simulink model "actuators_basicIO_2024a"  (R2024a)
settings: Solver=ode2  StartTime=0.0  StopTime=inf  FixedStep=1/500  RelTol=1e-3  EnableMultiTasking=on
undefined symbols (not defined in the file): HIL
libraries: quarc_library x85, simulink x4
settings Model: ExtModeTrigDuration=10000  Creator=Lorena Gonzalez  LastModifiedBy=Lorena Gonzalez
settings SolverCC: AlgebraicLoopSolver=TrustRegion  PositivePriorityOrder=on
settings DataIOCC: ReturnWorkspaceOutputs=off
settings DebuggingCC: UnconnectedInputMsg=warning  UnconnectedOutputMsg=warning  UnconnectedLineMsg=warning  ArithmeticOperatorsInVariantConditions=warning
settings ModelReferenceCC: EnableRefExpFcnMdlSchedulingChecks=on
settings SFSimCC: SimUseLocalCustomCode=off  CustomCodeUndefinedFunction=UseInterfaceOnly
settings RTWCC: Description=QUARC Win64 Target Using Toolchain  SystemTargetFile=quarc_win64.tlc  TemplateMakefile=quarc_default_tmf  RTWUseLocalCustomCode=off  Toolchain=QUARC win64 | nmake (64-bit Windows)  BuildConfiguration=Faster Runs  GPUComputeCapability=3.5
settings CodeAppCC: StateflowObjectComments=on
settings STFCustomTargetCC: ConcurrentExecutionCompliant=on  SystemTargetFile=quarc_win64.tlc
settings GRTTargetCC: ParMdlRefBuildCompliant=off  CompOptLevelCompliant=off  CombineOutputUpdateFcns=off  MatFileLogging=off  CPPClassGenCompliant=off  GRTInterface=on  ExtMode=on  ExtModeMexFile=quarc_comm
settings ConfigComp: CovMetricSettings=dswe

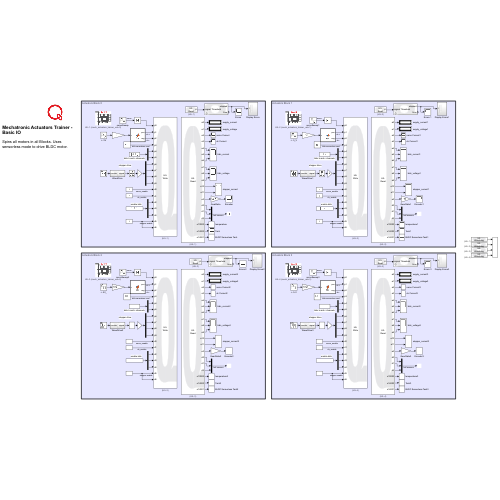
[thumbnail: Simulink's stored preview of the top-level diagram]
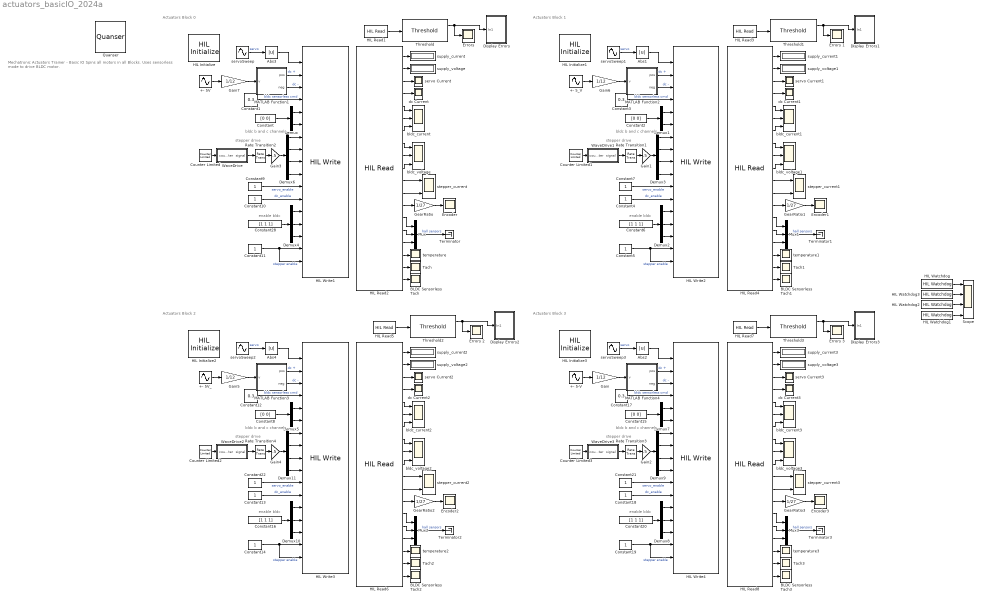
== system actuators_basicIO_2024a ==
  note: bldc b and c channels
  note: enable bldc
  note: Actuators Block 3
  note: Mechatronic Actuators Trainer - Basic IO
      |
      | Spins all motors in all Blocks. Uses sensorless mode to drive BLDC motor.
  note: bldc b and c channels
  note: stepper drive
  note: Actuators Block 0
  note: stepper drive
  note: Actuators Block 1
  note: enable bldc
  note: bldc b and c channels
  note: Actuators Block 2
  note: enable bldc
  note: stepper drive
  note: bldc b and c channels
  note: stepper drive
  note: enable bldc
  +- 5-V : Sin  Amplitude=5  Frequency=.75  SampleTime=0
  +- 5V : Sin  Amplitude=5  Frequency=.75  SampleTime=0
  +- 5V_ : Sin  Amplitude=5  Frequency=.75  SampleTime=0
  +- 5_V : Sin  Amplitude=5  Frequency=.75  SampleTime=0
  Abs{1..4} (4 alike) : Abs  SaturateOnIntegerOverflow=off
  BLDC Sensorless Tach{,1..3} (4 alike) : Scope
  Constant{,2,8,15} (4 alike) : Constant  Value=[0 0]
  Constant{1,3,12,17} (4 alike) : Constant  Value=0.3
  Constant{4..5,7,9..11,13..14,18..19,21..22} (12 alike) : Constant
  Constant{6,16,20,28} (4 alike) : Constant  Value=[1 1 1]
  Counter Limited{,1..3} (4 alike) : simulink/Sources/Counter Limited  uplimit=3  tsamp=1/100
  Demux{,1,5,7} (4 alike) : Demux  Outputs=2
  Demux{2,4,8,10} (4 alike) : Demux  Outputs=3
  Demux{3,6,9,11} (4 alike) : Demux
  Display Errors : Subsystem
  Display Errors1 : Subsystem
  Display Errors2 : Subsystem
  Display Errors3 : Subsystem
  Encoder{,1..3} (4 alike) : Scope
  Errors {,1..3} (4 alike) : Scope
  Gain{,5..7} (4 alike) : Gain  Gain=1/12
  Gain{1..4} (4 alike) : Gain  Gain=.5
  GearRatio{,1..3} (4 alike) : Gain  Gain=1/27
  HIL Initialize : quarc_library/Data Acquisition/Generic/Configuration/HIL Initialize  object_name=HIL-1  board_type=mech_actuators_trainer_usb  board_number=0  board_options=supply_voltage_low_limit=10.0;supply_voltage_high_limit=16.0;supply_current_high_limit=8.0;dc_motor_current_high_limit=1.1;servo_motor_current_high_limit=1.3;bldc_motor_current_high_limit=2.0;stepper_motor_current_high_limit=1.7;servo_pwm_range=0;enc_dir=0;bldc_motor_mode=1;bldc_start_tc=0.03;bldc_start_target=1200  exclusive=off  active=on  hardware_clocks=[0]  clock_modes=[]  initial_clock_frequencies=[]  set_clock_params_at_start=off  set_clock_params_at_switch_in=off  set_clock_frequencies_at_start=off  set_clock_frequencies_at_switch_in=off  analog_input_channels=[0:11]  analog_input_configurations=[]  analog_input_maximums=3  analog_input_minimums=-3  set_analog_input_params_at_start=off  set_analog_input_params_at_switch_in=off  analog_output_channels=[]  analog_output_maximums=[]  analog_output_minimums=[]  initial_analog_outputs=[]  final_analog_outputs=[]  watchdog_analog_outputs=[]  set_analog_output_params_at_start=off  set_analog_output_params_at_switch_in=off  set_analog_outputs_at_start=off  set_analog_outputs_at_switch_in=off  set_analog_outputs_at_terminate=off  set_analog_outputs_at_switch_out=off  set_analog_outputs_on_watchdog=off  digital_input_channels=[0:17]  digital_output_channels=[0:6]  digital_output_configuration=[]  initial_digital_outputs=[1]  final_digital_outputs=[0]  watchdog_digital_outputs=[0]  set_digital_output_params_at_start=off  set_digital_output_params_at_switch_in=off  set_digital_outputs_at_start=on  set_digital_outputs_at_switch_in=off  set_digital_outputs_at_terminate=on  set_digital_outputs_at_switch_out=off  set_digital_outputs_on_watchdog=on  encoder_channels=[0]  quadrature=[4]  encoder_filter_frequency=[]  initial_encoder_counts=[0]  set_encoder_params_at_start=on  set_encoder_params_at_switch_in=off  set_encoder_counts_at_start=on  set_encoder_counts_at_switch_in=off  pwm_channels=[0:9]  pwm_modes=[0]  pwm_frequency=23195  pwm_configuration=[1]  pwm_alignment=[0]  pwm_polarity=[1]  pwm_leading_deadband=[0]  pwm_trailing_deadband=[0]  initial_pwm_outputs=[0]  final_pwm_outputs=[0]  watchdog_pwm_outputs=[0]  set_pwm_params_at_start=off  set_pwm_params_at_switch_in=off  set_pwm_outputs_at_start=on  set_pwm_outputs_at_switch_in=off  set_pwm_outputs_at_terminate=on  set_pwm_outputs_at_switch_out=off  set_pwm_outputs_on_watchdog=on  other_output_channels=[]  initial_other_outputs=[]  final_other_outputs=[]  watchdog_other_outputs=[]  set_other_outputs_at_start=off  set_other_outputs_at_switch_in=off  set_other_outputs_at_terminate=off  set_other_outputs_at_switch_out=off  set_other_outputs_on_watchdog=off
  HIL Initialize1 : quarc_library/Data Acquisition/Generic/Configuration/HIL Initialize  object_name=HIL-2  board_type=mech_actuators_trainer_usb  board_number=1  board_options=supply_voltage_low_limit=10.0;supply_voltage_high_limit=16.0;supply_current_high_limit=8.0;dc_motor_current_high_limit=1.1;servo_motor_current_high_limit=1.3;bldc_motor_current_high_limit=2.0;stepper_motor_current_high_limit=1.7;servo_pwm_range=0;enc_dir=0;bldc_motor_mode=1;bldc_start_tc=0.03;bldc_start_target=1200  exclusive=off  active=on  hardware_clocks=[0]  clock_modes=[]  initial_clock_frequencies=[]  set_clock_params_at_start=off  set_clock_params_at_switch_in=off  set_clock_frequencies_at_start=off  set_clock_frequencies_at_switch_in=off  analog_input_channels=[0:11]  analog_input_configurations=[]  analog_input_maximums=3  analog_input_minimums=-3  set_analog_input_params_at_start=off  set_analog_input_params_at_switch_in=off  analog_output_channels=[]  analog_output_maximums=[]  analog_output_minimums=[]  initial_analog_outputs=[]  final_analog_outputs=[]  watchdog_analog_outputs=[]  set_analog_output_params_at_start=off  set_analog_output_params_at_switch_in=off  set_analog_outputs_at_start=off  set_analog_outputs_at_switch_in=off  set_analog_outputs_at_terminate=off  set_analog_outputs_at_switch_out=off  set_analog_outputs_on_watchdog=off  digital_input_channels=[0:17]  digital_output_channels=[0:6]  digital_output_configuration=[]  initial_digital_outputs=[1]  final_digital_outputs=[0]  watchdog_digital_outputs=[0]  set_digital_output_params_at_start=off  set_digital_output_params_at_switch_in=off  set_digital_outputs_at_start=on  set_digital_outputs_at_switch_in=off  set_digital_outputs_at_terminate=on  set_digital_outputs_at_switch_out=off  set_digital_outputs_on_watchdog=on  encoder_channels=[0]  quadrature=[4]  encoder_filter_frequency=[]  initial_encoder_counts=[0]  set_encoder_params_at_start=on  set_encoder_params_at_switch_in=off  set_encoder_counts_at_start=on  set_encoder_counts_at_switch_in=off  pwm_channels=[0:9]  pwm_modes=[0]  pwm_frequency=23195  pwm_configuration=[1]  pwm_alignment=[0]  pwm_polarity=[1]  pwm_leading_deadband=[0]  pwm_trailing_deadband=[0]  initial_pwm_outputs=[0]  final_pwm_outputs=[0]  watchdog_pwm_outputs=[0]  set_pwm_params_at_start=off  set_pwm_params_at_switch_in=off  set_pwm_outputs_at_start=on  set_pwm_outputs_at_switch_in=off  set_pwm_outputs_at_terminate=on  set_pwm_outputs_at_switch_out=off  set_pwm_outputs_on_watchdog=on  other_output_channels=[]  initial_other_outputs=[]  final_other_outputs=[]  watchdog_other_outputs=[]  set_other_outputs_at_start=off  set_other_outputs_at_switch_in=off  set_other_outputs_at_terminate=off  set_other_outputs_at_switch_out=off  set_other_outputs_on_watchdog=off
  HIL Initialize2 : quarc_library/Data Acquisition/Generic/Configuration/HIL Initialize  object_name=HIL-3  board_type=mech_actuators_trainer_usb  board_number=2  board_options=supply_voltage_low_limit=10.0;supply_voltage_high_limit=16.0;supply_current_high_limit=8.0;dc_motor_current_high_limit=1.1;servo_motor_current_high_limit=1.3;bldc_motor_current_high_limit=2.0;stepper_motor_current_high_limit=1.7;servo_pwm_range=0;enc_dir=0;bldc_motor_mode=1;bldc_start_tc=0.03;bldc_start_target=1200  exclusive=off  active=on  hardware_clocks=[0]  clock_modes=[]  initial_clock_frequencies=[]  set_clock_params_at_start=off  set_clock_params_at_switch_in=off  set_clock_frequencies_at_start=off  set_clock_frequencies_at_switch_in=off  analog_input_channels=[0:11]  analog_input_configurations=[]  analog_input_maximums=3  analog_input_minimums=-3  set_analog_input_params_at_start=off  set_analog_input_params_at_switch_in=off  analog_output_channels=[]  analog_output_maximums=[]  analog_output_minimums=[]  initial_analog_outputs=[]  final_analog_outputs=[]  watchdog_analog_outputs=[]  set_analog_output_params_at_start=off  set_analog_output_params_at_switch_in=off  set_analog_outputs_at_start=off  set_analog_outputs_at_switch_in=off  set_analog_outputs_at_terminate=off  set_analog_outputs_at_switch_out=off  set_analog_outputs_on_watchdog=off  digital_input_channels=[0:17]  digital_output_channels=[0:6]  digital_output_configuration=[]  initial_digital_outputs=[1]  final_digital_outputs=[0]  watchdog_digital_outputs=[0]  set_digital_output_params_at_start=off  set_digital_output_params_at_switch_in=off  set_digital_outputs_at_start=on  set_digital_outputs_at_switch_in=off  set_digital_outputs_at_terminate=on  set_digital_outputs_at_switch_out=off  set_digital_outputs_on_watchdog=on  encoder_channels=[0]  quadrature=[4]  encoder_filter_frequency=[]  initial_encoder_counts=[0]  set_encoder_params_at_start=on  set_encoder_params_at_switch_in=off  set_encoder_counts_at_start=on  set_encoder_counts_at_switch_in=off  pwm_channels=[0:9]  pwm_modes=[0]  pwm_frequency=23195  pwm_configuration=[1]  pwm_alignment=[0]  pwm_polarity=[1]  pwm_leading_deadband=[0]  pwm_trailing_deadband=[0]  initial_pwm_outputs=[0]  final_pwm_outputs=[0]  watchdog_pwm_outputs=[0]  set_pwm_params_at_start=off  set_pwm_params_at_switch_in=off  set_pwm_outputs_at_start=on  set_pwm_outputs_at_switch_in=off  set_pwm_outputs_at_terminate=on  set_pwm_outputs_at_switch_out=off  set_pwm_outputs_on_watchdog=on  other_output_channels=[]  initial_other_outputs=[]  final_other_outputs=[]  watchdog_other_outputs=[]  set_other_outputs_at_start=off  set_other_outputs_at_switch_in=off  set_other_outputs_at_terminate=off  set_other_outputs_at_switch_out=off  set_other_outputs_on_watchdog=off
  HIL Initialize3 : quarc_library/Data Acquisition/Generic/Configuration/HIL Initialize  object_name=HIL-4  board_type=mech_actuators_trainer_usb  board_number=3  board_options=supply_voltage_low_limit=10.0;supply_voltage_high_limit=16.0;supply_current_high_limit=8.0;dc_motor_current_high_limit=1.1;servo_motor_current_high_limit=1.3;bldc_motor_current_high_limit=2.0;stepper_motor_current_high_limit=1.7;servo_pwm_range=0;enc_dir=0;bldc_motor_mode=1;bldc_start_tc=0.03;bldc_start_target=1200  exclusive=off  active=on  hardware_clocks=[0]  clock_modes=[]  initial_clock_frequencies=[]  set_clock_params_at_start=off  set_clock_params_at_switch_in=off  set_clock_frequencies_at_start=off  set_clock_frequencies_at_switch_in=off  analog_input_channels=[0:11]  analog_input_configurations=[]  analog_input_maximums=3  analog_input_minimums=-3  set_analog_input_params_at_start=off  set_analog_input_params_at_switch_in=off  analog_output_channels=[]  analog_output_maximums=[]  analog_output_minimums=[]  initial_analog_outputs=[]  final_analog_outputs=[]  watchdog_analog_outputs=[]  set_analog_output_params_at_start=off  set_analog_output_params_at_switch_in=off  set_analog_outputs_at_start=off  set_analog_outputs_at_switch_in=off  set_analog_outputs_at_terminate=off  set_analog_outputs_at_switch_out=off  set_analog_outputs_on_watchdog=off  digital_input_channels=[0:17]  digital_output_channels=[0:6]  digital_output_configuration=[]  initial_digital_outputs=[1]  final_digital_outputs=[0]  watchdog_digital_outputs=[0]  set_digital_output_params_at_start=off  set_digital_output_params_at_switch_in=off  set_digital_outputs_at_start=on  set_digital_outputs_at_switch_in=off  set_digital_outputs_at_terminate=on  set_digital_outputs_at_switch_out=off  set_digital_outputs_on_watchdog=on  encoder_channels=[0]  quadrature=[4]  encoder_filter_frequency=[]  initial_encoder_counts=[0]  set_encoder_params_at_start=on  set_encoder_params_at_switch_in=off  set_encoder_counts_at_start=on  set_encoder_counts_at_switch_in=off  pwm_channels=[0:9]  pwm_modes=[0]  pwm_frequency=23195  pwm_configuration=[1]  pwm_alignment=[0]  pwm_polarity=[1]  pwm_leading_deadband=[0]  pwm_trailing_deadband=[0]  initial_pwm_outputs=[0]  final_pwm_outputs=[0]  watchdog_pwm_outputs=[0]  set_pwm_params_at_start=off  set_pwm_params_at_switch_in=off  set_pwm_outputs_at_start=on  set_pwm_outputs_at_switch_in=off  set_pwm_outputs_at_terminate=on  set_pwm_outputs_at_switch_out=off  set_pwm_outputs_on_watchdog=on  other_output_channels=[]  initial_other_outputs=[]  final_other_outputs=[]  watchdog_other_outputs=[]  set_other_outputs_at_start=off  set_other_outputs_at_switch_in=off  set_other_outputs_at_terminate=off  set_other_outputs_at_switch_out=off  set_other_outputs_on_watchdog=off
  HIL Read1 : quarc_library/Data Acquisition/Generic/Immediate I//O/HIL Read  object_name=HIL-1  analog_channels=[]  encoder_channels=[]  digital_channels=[3:17]  other_channels=[]  sample_time=qc_get_step_size  active=on  vector_output=on  data_type_mode=Inherit via back propagation  encoder_data_type=double  digital_data_type=boolean
  HIL Read2 : quarc_library/Data Acquisition/Generic/Immediate I//O/HIL Read  object_name=HIL-1  analog_channels=[0:11]  encoder_channels=[0]  digital_channels=[0:2]  other_channels=[10000 14000:14001]  sample_time=qc_get_step_size  active=on  vector_output=off  data_type_mode=Inherit via back propagation  encoder_data_type=double  digital_data_type=boolean
  HIL Read3 : quarc_library/Data Acquisition/Generic/Immediate I//O/HIL Read  object_name=HIL-2  analog_channels=[]  encoder_channels=[]  digital_channels=[3:17]  other_channels=[]  sample_time=qc_get_step_size  active=on  vector_output=on  data_type_mode=Inherit via back propagation  encoder_data_type=double  digital_data_type=boolean
  HIL Read4 : quarc_library/Data Acquisition/Generic/Immediate I//O/HIL Read  object_name=HIL-2  analog_channels=[0:11]  encoder_channels=[0]  digital_channels=[0:2]  other_channels=[10000 14000:14001]  sample_time=qc_get_step_size  active=on  vector_output=off  data_type_mode=Inherit via back propagation  encoder_data_type=double  digital_data_type=boolean
  HIL Read5 : quarc_library/Data Acquisition/Generic/Immediate I//O/HIL Read  object_name=HIL-3  analog_channels=[]  encoder_channels=[]  digital_channels=[3:17]  other_channels=[]  sample_time=qc_get_step_size  active=on  vector_output=on  data_type_mode=Inherit via back propagation  encoder_data_type=double  digital_data_type=boolean
  HIL Read6 : quarc_library/Data Acquisition/Generic/Immediate I//O/HIL Read  object_name=HIL-3  analog_channels=[0:11]  encoder_channels=[0]  digital_channels=[0:2]  other_channels=[10000 14000:14001]  sample_time=qc_get_step_size  active=on  vector_output=off  data_type_mode=Inherit via back propagation  encoder_data_type=double  digital_data_type=boolean
  HIL Read7 : quarc_library/Data Acquisition/Generic/Immediate I//O/HIL Read  object_name=HIL-4  analog_channels=[]  encoder_channels=[]  digital_channels=[3:17]  other_channels=[]  sample_time=qc_get_step_size  active=on  vector_output=on  data_type_mode=Inherit via back propagation  encoder_data_type=double  digital_data_type=boolean
  HIL Read8 : quarc_library/Data Acquisition/Generic/Immediate I//O/HIL Read  object_name=HIL-4  analog_channels=[0:11]  encoder_channels=[0]  digital_channels=[0:2]  other_channels=[10000 14000:14001]  sample_time=qc_get_step_size  active=on  vector_output=off  data_type_mode=Inherit via back propagation  encoder_data_type=double  digital_data_type=boolean
  HIL Watchdog : quarc_library/Data Acquisition/Generic/Watchdog/HIL Watchdog  object_name=HIL-1  timeout=0.1  sample_time=qc_get_step_size  active=off
      settings: AttributesFormatString=(%<object_name>)  SourceProductName=QUARC Targets
  HIL Watchdog1 : quarc_library/Data Acquisition/Generic/Watchdog/HIL Watchdog  object_name=HIL-4  timeout=0.1  sample_time=qc_get_step_size  active=off
      settings: AttributesFormatString=(%<object_name>)  SourceProductName=QUARC Targets
  HIL Watchdog2 : quarc_library/Data Acquisition/Generic/Watchdog/HIL Watchdog  object_name=HIL-3  timeout=0.1  sample_time=qc_get_step_size  active=off
      settings: AttributesFormatString=(%<object_name>)  SourceProductName=QUARC Targets
  HIL Watchdog3 : quarc_library/Data Acquisition/Generic/Watchdog/HIL Watchdog  object_name=HIL-2  timeout=0.1  sample_time=qc_get_step_size  active=off
      settings: AttributesFormatString=(%<object_name>)  SourceProductName=QUARC Targets
  HIL Write1 : quarc_library/Data Acquisition/Generic/Immediate I//O/HIL Write  object_name=HIL-1  analog_channels=[]  pwm_channels=[0:9]  digital_channels=[0:6]  other_channels=[]  sample_time=-1  active=off  vector_input=off
  HIL Write2 : quarc_library/Data Acquisition/Generic/Immediate I//O/HIL Write  object_name=HIL-2  analog_channels=[]  pwm_channels=[0:9]  digital_channels=[0:6]  other_channels=[]  sample_time=-1  active=off  vector_input=off
  HIL Write3 : quarc_library/Data Acquisition/Generic/Immediate I//O/HIL Write  object_name=HIL-3  analog_channels=[]  pwm_channels=[0:9]  digital_channels=[0:6]  other_channels=[]  sample_time=-1  active=off  vector_input=off
  HIL Write4 : quarc_library/Data Acquisition/Generic/Immediate I//O/HIL Write  object_name=HIL-4  analog_channels=[]  pwm_channels=[0:9]  digital_channels=[0:6]  other_channels=[]  sample_time=-1  active=off  vector_input=off
  MATLAB Function1 : MATLAB Function  TreatAsAtomicUnit=on
  MATLAB Function2 : MATLAB Function  TreatAsAtomicUnit=on
  MATLAB Function3 : MATLAB Function  TreatAsAtomicUnit=on
  MATLAB Function4 : MATLAB Function  TreatAsAtomicUnit=on
  Mux{,1..3} (4 alike) : Mux  Inputs=3
  Quanser : quarc_library/Logos/Quanser
  Rate Transition{1..4} (4 alike) : RateTransition
  Scope : Scope  NumInputPorts=4
  Tach{,1..3} (4 alike) : Scope
  Terminator{,1..3} (4 alike) : Terminator
  Threshold{,1..3} (4 alike) : quarc_library/Discontinuities/Threshold  operator=>  param_src=Specify via dialog  threshold=0  duration=0.02
      settings: SourceProductName=QUARC Targets
  WaveDrive : Subsystem
  WaveDrive1 : Subsystem
  WaveDrive2 : Subsystem
  WaveDrive3 : Subsystem
  bldc_current{,1..3} (4 alike) : Scope  NumInputPorts=3
  bldc_voltage{,1..3} (4 alike) : Scope  NumInputPorts=3
  dc Current{,1..3} (4 alike) : Scope
  servo Current{,1..3} (4 alike) : Scope
  servoSweep{,1..3} (4 alike) : Sin  SampleTime=0
  stepper_current{,1..3} (4 alike) : Scope  NumInputPorts=2
  supply_current{,1..3} (4 alike) : Display
  supply_voltage{,1..3} (4 alike) : Display
  temperature{,1..3} (4 alike) : Scope
  wires:
  Demux10/3 -> HIL Write3/15
  Demux11/4 -> HIL Write3/10
  HIL Read7/1 -> Threshold3/1
  HIL Read6/1 -> supply_current2/1
  HIL Read8/12 -> stepper_current3/2
  Threshold3/1 -> Display Errors3/1(In1), Errors 3/1
  HIL Read8/3 -> servo Current3/1
  HIL Read8/10 -> bldc_voltage3/3
  Rate Transition2/1 -> Gain3/1
  MATLAB Function2/2(neg) -> HIL Write2/3  "dc -"
  Gain5/1 -> MATLAB Function3/1(v)
  HIL Read8/6 -> bldc_current3/2
  HIL Read3/1 -> Threshold1/1
  HIL Read6/19 -> BLDC Sensorless Tach2/1
  HIL Read6/10 -> bldc_voltage2/3
  HIL Read5/1 -> Threshold2/1
  HIL Read4/11 -> stepper_current1/1
  Threshold1/1 -> Display Errors1/1(In1), Errors 1/1
  Threshold2/1 -> Display Errors2/1(In1), Errors 2/1
  HIL Read1/1 -> Threshold/1
  GearRatio1/1 -> Encoder1/1
  Counter Limited3/1 -> WaveDrive3/1(counter)
  Demux6/4 -> HIL Write1/10
  Constant5/1 -> HIL Write2/16, HIL Write2/17  "stepper enable"
  servoSweep2/1 -> Abs4/1  "servo"
  GearRatio3/1 -> Encoder3/1
  Constant7/1 -> HIL Write2/11  "servo_enable"
  HIL Read2/7 -> bldc_current/3
  Constant/1 -> Demux/1
  Demux9/3 -> HIL Write4/9
  Gain7/1 -> MATLAB Function1/1(v)
  Gain/1 -> MATLAB Function4/1(v)
  Demux11/2 -> HIL Write3/8
  Demux8/2 -> HIL Write4/14
  HIL Read2/11 -> stepper_current/1
  Counter Limited/1 -> WaveDrive/1(counter)
  HIL Read6/3 -> servo Current2/1
  HIL Read6/16 -> Mux2/3
  WaveDrive2/1(signal) -> Rate Transition4/1
  HIL Read8/19 -> BLDC Sensorless Tach3/1
  HIL Read8/9 -> bldc_voltage3/2
  Constant14/1 -> HIL Write3/16, HIL Write3/17  "stepper enable"
  Constant8/1 -> Demux5/1
  Demux10/2 -> HIL Write3/14
  HIL Read8/16 -> Mux3/3
  Constant13/1 -> HIL Write3/12  "dc_enable"
  HIL Read6/11 -> stepper_current2/1
  HIL Read6/12 -> stepper_current2/2
  Demux8/1 -> HIL Write4/13
  Constant10/1 -> HIL Write1/12  "dc_enable"
  HIL Read6/18 -> Tach2/1
  Constant22/1 -> HIL Write3/11  "servo_enable"
  Demux11/1 -> HIL Write3/7
  Constant15/1 -> Demux7/1
  HIL Read6/4 -> dc Current2/1
  MATLAB Function3/1(pos) -> HIL Write3/2  "dc +"
  HIL Read6/6 -> bldc_current2/2
  HIL Read4/12 -> stepper_current1/2
  Mux1/1 -> Terminator1/1  "hall sensors"
  Mux2/1 -> Terminator2/1  "hall sensors"
  HIL Read6/9 -> bldc_voltage2/2
  HIL Read6/7 -> bldc_current2/3
  HIL Read6/2 -> supply_voltage2/1
  Rate Transition4/1 -> Gain4/1
  Demux7/1 -> HIL Write4/5
  Demux8/3 -> HIL Write4/15
  Demux6/1 -> HIL Write1/7
  MATLAB Function2/1(pos) -> HIL Write2/2  "dc +"
  Gain4/1 -> Demux11/1
  Mux3/1 -> Terminator3/1  "hall sensors"
  HIL Read6/8 -> bldc_voltage2/1
  Demux9/4 -> HIL Write4/10
  MATLAB Function3/2(neg) -> HIL Write3/3  "dc -"
  Counter Limited1/1 -> WaveDrive1/1(counter)
  servoSweep1/1 -> Abs1/1  "servo"
  GearRatio2/1 -> Encoder2/1
  Counter Limited2/1 -> WaveDrive2/1(counter)
  HIL Read8/17 -> temperature3/1
  Demux/1 -> HIL Write1/5
  Gain2/1 -> Demux9/1
  servoSweep3/1 -> Abs2/1  "servo"
  HIL Read6/5 -> bldc_current2/1
  WaveDrive1/1(signal) -> Rate Transition1/1
  HIL Read4/16 -> Mux1/3
  Constant1/1 -> HIL Write1/4  "bldc sensorless cmd"
  Demux10/1 -> HIL Write3/13
  Abs4/1 -> HIL Write3/1
  HIL Read2/1 -> supply_current/1
  Constant12/1 -> HIL Write3/4  "bldc sensorless cmd"
  Constant16/1 -> Demux10/1
  Abs2/1 -> HIL Write4/1
  HIL Read6/17 -> temperature2/1
  Demux5/1 -> HIL Write3/5
  HIL Read4/8 -> bldc_voltage1/1
  Constant20/1 -> Demux8/1
  HIL Read8/13 -> GearRatio3/1
  WaveDrive3/1(signal) -> Rate Transition3/1
  HIL Read6/15 -> Mux2/2
  HIL Read4/3 -> servo Current1/1
  Rate Transition3/1 -> Gain2/1
  Demux7/2 -> HIL Write4/6
  HIL Read8/14 -> Mux3/1
  Demux9/1 -> HIL Write4/7
  Gain1/1 -> Demux3/1
  MATLAB Function4/1(pos) -> HIL Write4/2  "dc +"
  HIL Read8/7 -> bldc_current3/3
  Constant17/1 -> HIL Write4/4  "bldc sensorless cmd"
  HIL Read2/5 -> bldc_current/1
  Constant21/1 -> HIL Write4/11  "servo_enable"
  Demux9/2 -> HIL Write4/8
  HIL Read8/18 -> Tach3/1
  HIL Read8/4 -> dc Current3/1
  HIL Read8/8 -> bldc_voltage3/1
  HIL Read4/19 -> BLDC Sensorless Tach1/1
  Constant19/1 -> HIL Write4/16, HIL Write4/17  "stepper enable"
  HIL Read8/2 -> supply_voltage3/1
  HIL Read4/2 -> supply_voltage1/1
  HIL Read8/15 -> Mux3/2
  HIL Read4/18 -> Tach1/1
  HIL Read4/6 -> bldc_current1/2
  HIL Read4/14 -> Mux1/1
  Constant4/1 -> HIL Write2/12  "dc_enable"
  Demux2/1 -> HIL Write2/13
  HIL Read2/6 -> bldc_current/2
  HIL Read8/1 -> supply_current3/1
  HIL Read4/10 -> bldc_voltage1/3
  Rate Transition1/1 -> Gain1/1
  Demux1/2 -> HIL Write2/6
  HIL Read4/7 -> bldc_current1/3
  Demux2/2 -> HIL Write2/14
  HIL Read2/14 -> Mux/1
  Constant2/1 -> Demux1/1
  Demux11/3 -> HIL Write3/9
  HIL Read4/1 -> supply_current1/1
  MATLAB Function4/2(neg) -> HIL Write4/3  "dc -"
  HIL Read4/13 -> GearRatio1/1
  Gain6/1 -> MATLAB Function2/1(v)
  HIL Read6/14 -> Mux2/1
  Demux3/4 -> HIL Write2/10
  HIL Read4/9 -> bldc_voltage1/2
  Abs1/1 -> HIL Write2/1
  Demux4/3 -> HIL Write1/15
  Constant3/1 -> HIL Write2/4  "bldc sensorless cmd"
  HIL Read2/16 -> Mux/3
  Demux3/3 -> HIL Write2/9
  HIL Read2/19 -> BLDC Sensorless Tach/1
  HIL Read4/15 -> Mux1/2
  +- 5V_/1 -> Gain5/1
  Demux/2 -> HIL Write1/6
  MATLAB Function1/1(pos) -> HIL Write1/2  "dc +"
  Demux3/2 -> HIL Write2/8
  HIL Read6/13 -> GearRatio2/1
  HIL Read2/13 -> GearRatio/1
  HIL Watchdog3/1 -> Scope/2
  Demux1/1 -> HIL Write2/5
  HIL Read2/9 -> bldc_voltage/2
  Demux2/3 -> HIL Write2/15
  HIL Watchdog/1 -> Scope/1
  +- 5_V/1 -> Gain6/1
  HIL Read2/8 -> bldc_voltage/1
  HIL Watchdog1/1 -> Scope/4
  Mux/1 -> Terminator/1  "hall sensors"
  HIL Read2/15 -> Mux/2
  HIL Read2/10 -> bldc_voltage/3
  Demux3/1 -> HIL Write2/7
  Constant28/1 -> Demux4/1
  servoSweep/1 -> Abs3/1  "servo"
  HIL Watchdog2/1 -> Scope/3
  HIL Read2/17 -> temperature/1
  HIL Read2/2 -> supply_voltage/1
  MATLAB Function1/2(neg) -> HIL Write1/3  "dc -"
  HIL Read8/11 -> stepper_current3/1
  Demux4/1 -> HIL Write1/13
  WaveDrive/1(signal) -> Rate Transition2/1
  HIL Read4/5 -> bldc_current1/1
  Abs3/1 -> HIL Write1/1
  Constant18/1 -> HIL Write4/12  "dc_enable"
  Demux6/3 -> HIL Write1/9
  +- 5-V/1 -> Gain/1
  Gain3/1 -> Demux6/1
  Constant6/1 -> Demux2/1
  HIL Read2/3 -> servo Current/1
  +- 5V/1 -> Gain7/1
  Demux5/2 -> HIL Write3/6
  HIL Read4/17 -> temperature1/1
  Demux6/2 -> HIL Write1/8
  HIL Read8/5 -> bldc_current3/1
  Constant9/1 -> HIL Write1/11  "servo_enable"
  Constant11/1 -> HIL Write1/16, HIL Write1/17  "stepper enable"
  HIL Read2/12 -> stepper_current/2
  HIL Read2/18 -> Tach/1
  Demux4/2 -> HIL Write1/14
  Threshold/1 -> Display Errors/1(In1), "Errors "/1
  HIL Read2/4 -> dc Current/1
  GearRatio/1 -> Encoder/1
  HIL Read4/4 -> dc Current1/1

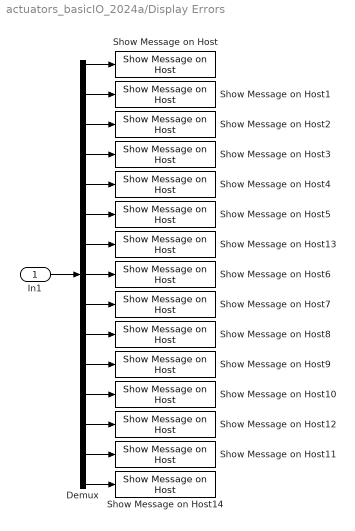
== system actuators_basicIO_2024a/Display Errors ==
  In1 : Inport
  Demux : Demux  Outputs=15
  Show Message on Host : quarc_library/Sinks/Error Handling/Show Message on Host  message_type=Fixed error message  message_icon=Error  message=Power Supply Voltage Too Low
      settings: AttributesFormatString="\"%<message>\""  SourceProductName=QUARC Targets
  Show Message on Host1 : quarc_library/Sinks/Error Handling/Show Message on Host  message_type=Fixed error message  message_icon=Error  message=Power Supply Voltage Too High
      settings: AttributesFormatString="\"%<message>\""  SourceProductName=QUARC Targets
  Show Message on Host10 : quarc_library/Sinks/Error Handling/Show Message on Host  message_type=Fixed error message  message_icon=Error  message=Stepper Channel B Current Too High
      settings: AttributesFormatString="\"%<message>\""  SourceProductName=QUARC Targets
  Show Message on Host11 : quarc_library/Sinks/Error Handling/Show Message on Host  message_type=Fixed error message  message_icon=Error  message=Stepper Channel B Driver Over Current/Temperature
      settings: AttributesFormatString="\"%<message>\""  SourceProductName=QUARC Targets
  Show Message on Host12 : quarc_library/Sinks/Error Handling/Show Message on Host  message_type=Fixed error message  message_icon=Error  message=Stepper Channel A Driver Over Current/Temperature
      settings: AttributesFormatString="\"%<message>\""  SourceProductName=QUARC Targets
  Show Message on Host13 : quarc_library/Sinks/Error Handling/Show Message on Host  message_type=Fixed error message  message_icon=Error  message=Servo Motor Voltage Out of Range
      settings: AttributesFormatString="\"%<message>\""  SourceProductName=QUARC Targets
  Show Message on Host14 : quarc_library/Sinks/Error Handling/Show Message on Host  message_type=Fixed error message  message_icon=Error  message=Device Over-Temperature
      settings: AttributesFormatString="\"%<message>\""  SourceProductName=QUARC Targets
  Show Message on Host2 : quarc_library/Sinks/Error Handling/Show Message on Host  message_type=Fixed error message  message_icon=Error  message=Power Supply Current Too High
      settings: AttributesFormatString="\"%<message>\""  SourceProductName=QUARC Targets
  Show Message on Host3 : quarc_library/Sinks/Error Handling/Show Message on Host  message_type=Fixed error message  message_icon=Error  message=DC Motor Current Too High
      settings: AttributesFormatString="\"%<message>\""  SourceProductName=QUARC Targets
  Show Message on Host4 : quarc_library/Sinks/Error Handling/Show Message on Host  message_type=Fixed error message  message_icon=Error  message=DC Motor Driver Over Current/Temperature
      settings: AttributesFormatString="\"%<message>\""  SourceProductName=QUARC Targets
  Show Message on Host5 : quarc_library/Sinks/Error Handling/Show Message on Host  message_type=Fixed error message  message_icon=Error  message=Servo Motor Current Too High
      settings: AttributesFormatString="\"%<message>\""  SourceProductName=QUARC Targets
  Show Message on Host6 : quarc_library/Sinks/Error Handling/Show Message on Host  message_type=Fixed error message  message_icon=Error  message=BLDC Channel A Current Too High
      settings: AttributesFormatString="\"%<message>\""  SourceProductName=QUARC Targets
  Show Message on Host7 : quarc_library/Sinks/Error Handling/Show Message on Host  message_type=Fixed error message  message_icon=Error  message=BLDC Channel B Current Too High
      settings: AttributesFormatString="\"%<message>\""  SourceProductName=QUARC Targets
  Show Message on Host8 : quarc_library/Sinks/Error Handling/Show Message on Host  message_type=Fixed error message  message_icon=Error  message=BLDC Channel C Current Too High
      settings: AttributesFormatString="\"%<message>\""  SourceProductName=QUARC Targets
  Show Message on Host9 : quarc_library/Sinks/Error Handling/Show Message on Host  message_type=Fixed error message  message_icon=Error  message=Stepper Channel A Current Too High
      settings: AttributesFormatString="\"%<message>\""  SourceProductName=QUARC Targets
  wires:
  In1/1 -> Demux/1
  Demux/1 -> Show Message on Host/1
  Demux/2 -> Show Message on Host1/1
  Demux/3 -> Show Message on Host2/1
  Demux/4 -> Show Message on Host3/1
  Demux/5 -> Show Message on Host4/1
  Demux/6 -> Show Message on Host5/1
  Demux/8 -> Show Message on Host6/1
  Demux/9 -> Show Message on Host7/1
  Demux/10 -> Show Message on Host8/1
  Demux/11 -> Show Message on Host9/1
  Demux/12 -> Show Message on Host10/1
  Demux/13 -> Show Message on Host12/1
  Demux/14 -> Show Message on Host11/1
  Demux/15 -> Show Message on Host14/1
  Demux/7 -> Show Message on Host13/1

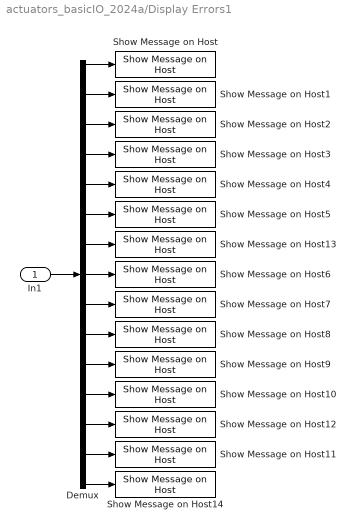
== system actuators_basicIO_2024a/Display Errors1 ==
  In1 : Inport
  Demux : Demux  Outputs=15
  Show Message on Host : quarc_library/Sinks/Error Handling/Show Message on Host  message_type=Fixed error message  message_icon=Error  message=Power Supply Voltage Too Low
      settings: AttributesFormatString="\"%<message>\""  SourceProductName=QUARC Targets
  Show Message on Host1 : quarc_library/Sinks/Error Handling/Show Message on Host  message_type=Fixed error message  message_icon=Error  message=Power Supply Voltage Too High
      settings: AttributesFormatString="\"%<message>\""  SourceProductName=QUARC Targets
  Show Message on Host10 : quarc_library/Sinks/Error Handling/Show Message on Host  message_type=Fixed error message  message_icon=Error  message=Stepper Channel B Current Too High
      settings: AttributesFormatString="\"%<message>\""  SourceProductName=QUARC Targets
  Show Message on Host11 : quarc_library/Sinks/Error Handling/Show Message on Host  message_type=Fixed error message  message_icon=Error  message=Stepper Channel B Driver Over Current/Temperature
      settings: AttributesFormatString="\"%<message>\""  SourceProductName=QUARC Targets
  Show Message on Host12 : quarc_library/Sinks/Error Handling/Show Message on Host  message_type=Fixed error message  message_icon=Error  message=Stepper Channel A Driver Over Current/Temperature
      settings: AttributesFormatString="\"%<message>\""  SourceProductName=QUARC Targets
  Show Message on Host13 : quarc_library/Sinks/Error Handling/Show Message on Host  message_type=Fixed error message  message_icon=Error  message=Servo Motor Voltage Out of Range
      settings: AttributesFormatString="\"%<message>\""  SourceProductName=QUARC Targets
  Show Message on Host14 : quarc_library/Sinks/Error Handling/Show Message on Host  message_type=Fixed error message  message_icon=Error  message=Device Over-Temperature
      settings: AttributesFormatString="\"%<message>\""  SourceProductName=QUARC Targets
  Show Message on Host2 : quarc_library/Sinks/Error Handling/Show Message on Host  message_type=Fixed error message  message_icon=Error  message=Power Supply Current Too High
      settings: AttributesFormatString="\"%<message>\""  SourceProductName=QUARC Targets
  Show Message on Host3 : quarc_library/Sinks/Error Handling/Show Message on Host  message_type=Fixed error message  message_icon=Error  message=DC Motor Current Too High
      settings: AttributesFormatString="\"%<message>\""  SourceProductName=QUARC Targets
  Show Message on Host4 : quarc_library/Sinks/Error Handling/Show Message on Host  message_type=Fixed error message  message_icon=Error  message=DC Motor Driver Over Current/Temperature
      settings: AttributesFormatString="\"%<message>\""  SourceProductName=QUARC Targets
  Show Message on Host5 : quarc_library/Sinks/Error Handling/Show Message on Host  message_type=Fixed error message  message_icon=Error  message=Servo Motor Current Too High
      settings: AttributesFormatString="\"%<message>\""  SourceProductName=QUARC Targets
  Show Message on Host6 : quarc_library/Sinks/Error Handling/Show Message on Host  message_type=Fixed error message  message_icon=Error  message=BLDC Channel A Current Too High
      settings: AttributesFormatString="\"%<message>\""  SourceProductName=QUARC Targets
  Show Message on Host7 : quarc_library/Sinks/Error Handling/Show Message on Host  message_type=Fixed error message  message_icon=Error  message=BLDC Channel B Current Too High
      settings: AttributesFormatString="\"%<message>\""  SourceProductName=QUARC Targets
  Show Message on Host8 : quarc_library/Sinks/Error Handling/Show Message on Host  message_type=Fixed error message  message_icon=Error  message=BLDC Channel C Current Too High
      settings: AttributesFormatString="\"%<message>\""  SourceProductName=QUARC Targets
  Show Message on Host9 : quarc_library/Sinks/Error Handling/Show Message on Host  message_type=Fixed error message  message_icon=Error  message=Stepper Channel A Current Too High
      settings: AttributesFormatString="\"%<message>\""  SourceProductName=QUARC Targets
  wires:
  In1/1 -> Demux/1
  Demux/1 -> Show Message on Host/1
  Demux/2 -> Show Message on Host1/1
  Demux/3 -> Show Message on Host2/1
  Demux/4 -> Show Message on Host3/1
  Demux/5 -> Show Message on Host4/1
  Demux/6 -> Show Message on Host5/1
  Demux/8 -> Show Message on Host6/1
  Demux/9 -> Show Message on Host7/1
  Demux/10 -> Show Message on Host8/1
  Demux/11 -> Show Message on Host9/1
  Demux/12 -> Show Message on Host10/1
  Demux/13 -> Show Message on Host12/1
  Demux/14 -> Show Message on Host11/1
  Demux/15 -> Show Message on Host14/1
  Demux/7 -> Show Message on Host13/1

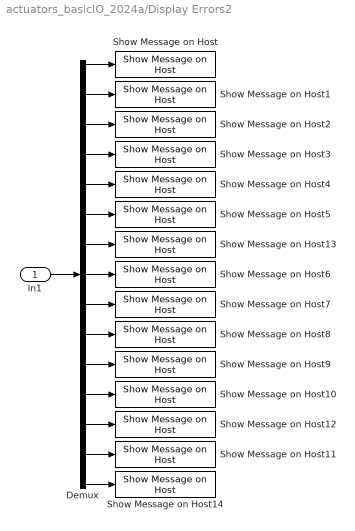
== system actuators_basicIO_2024a/Display Errors2 ==
  In1 : Inport
  Demux : Demux  Outputs=15
  Show Message on Host : quarc_library/Sinks/Error Handling/Show Message on Host  message_type=Fixed error message  message_icon=Error  message=Power Supply Voltage Too Low
      settings: AttributesFormatString="\"%<message>\""  SourceProductName=QUARC Targets
  Show Message on Host1 : quarc_library/Sinks/Error Handling/Show Message on Host  message_type=Fixed error message  message_icon=Error  message=Power Supply Voltage Too High
      settings: AttributesFormatString="\"%<message>\""  SourceProductName=QUARC Targets
  Show Message on Host10 : quarc_library/Sinks/Error Handling/Show Message on Host  message_type=Fixed error message  message_icon=Error  message=Stepper Channel B Current Too High
      settings: AttributesFormatString="\"%<message>\""  SourceProductName=QUARC Targets
  Show Message on Host11 : quarc_library/Sinks/Error Handling/Show Message on Host  message_type=Fixed error message  message_icon=Error  message=Stepper Channel B Driver Over Current/Temperature
      settings: AttributesFormatString="\"%<message>\""  SourceProductName=QUARC Targets
  Show Message on Host12 : quarc_library/Sinks/Error Handling/Show Message on Host  message_type=Fixed error message  message_icon=Error  message=Stepper Channel A Driver Over Current/Temperature
      settings: AttributesFormatString="\"%<message>\""  SourceProductName=QUARC Targets
  Show Message on Host13 : quarc_library/Sinks/Error Handling/Show Message on Host  message_type=Fixed error message  message_icon=Error  message=Servo Motor Voltage Out of Range
      settings: AttributesFormatString="\"%<message>\""  SourceProductName=QUARC Targets
  Show Message on Host14 : quarc_library/Sinks/Error Handling/Show Message on Host  message_type=Fixed error message  message_icon=Error  message=Device Over-Temperature
      settings: AttributesFormatString="\"%<message>\""  SourceProductName=QUARC Targets
  Show Message on Host2 : quarc_library/Sinks/Error Handling/Show Message on Host  message_type=Fixed error message  message_icon=Error  message=Power Supply Current Too High
      settings: AttributesFormatString="\"%<message>\""  SourceProductName=QUARC Targets
  Show Message on Host3 : quarc_library/Sinks/Error Handling/Show Message on Host  message_type=Fixed error message  message_icon=Error  message=DC Motor Current Too High
      settings: AttributesFormatString="\"%<message>\""  SourceProductName=QUARC Targets
  Show Message on Host4 : quarc_library/Sinks/Error Handling/Show Message on Host  message_type=Fixed error message  message_icon=Error  message=DC Motor Driver Over Current/Temperature
      settings: AttributesFormatString="\"%<message>\""  SourceProductName=QUARC Targets
  Show Message on Host5 : quarc_library/Sinks/Error Handling/Show Message on Host  message_type=Fixed error message  message_icon=Error  message=Servo Motor Current Too High
      settings: AttributesFormatString="\"%<message>\""  SourceProductName=QUARC Targets
  Show Message on Host6 : quarc_library/Sinks/Error Handling/Show Message on Host  message_type=Fixed error message  message_icon=Error  message=BLDC Channel A Current Too High
      settings: AttributesFormatString="\"%<message>\""  SourceProductName=QUARC Targets
  Show Message on Host7 : quarc_library/Sinks/Error Handling/Show Message on Host  message_type=Fixed error message  message_icon=Error  message=BLDC Channel B Current Too High
      settings: AttributesFormatString="\"%<message>\""  SourceProductName=QUARC Targets
  Show Message on Host8 : quarc_library/Sinks/Error Handling/Show Message on Host  message_type=Fixed error message  message_icon=Error  message=BLDC Channel C Current Too High
      settings: AttributesFormatString="\"%<message>\""  SourceProductName=QUARC Targets
  Show Message on Host9 : quarc_library/Sinks/Error Handling/Show Message on Host  message_type=Fixed error message  message_icon=Error  message=Stepper Channel A Current Too High
      settings: AttributesFormatString="\"%<message>\""  SourceProductName=QUARC Targets
  wires:
  In1/1 -> Demux/1
  Demux/1 -> Show Message on Host/1
  Demux/2 -> Show Message on Host1/1
  Demux/3 -> Show Message on Host2/1
  Demux/4 -> Show Message on Host3/1
  Demux/5 -> Show Message on Host4/1
  Demux/6 -> Show Message on Host5/1
  Demux/8 -> Show Message on Host6/1
  Demux/9 -> Show Message on Host7/1
  Demux/10 -> Show Message on Host8/1
  Demux/11 -> Show Message on Host9/1
  Demux/12 -> Show Message on Host10/1
  Demux/13 -> Show Message on Host12/1
  Demux/14 -> Show Message on Host11/1
  Demux/15 -> Show Message on Host14/1
  Demux/7 -> Show Message on Host13/1

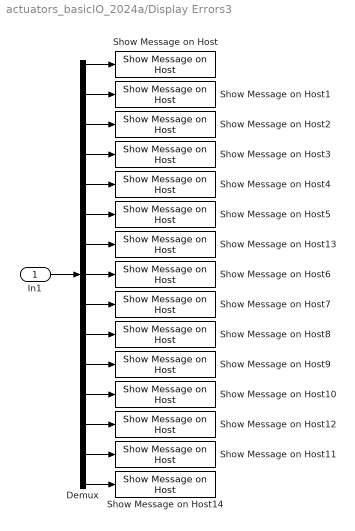
== system actuators_basicIO_2024a/Display Errors3 ==
  In1 : Inport
  Demux : Demux  Outputs=15
  Show Message on Host : quarc_library/Sinks/Error Handling/Show Message on Host  message_type=Fixed error message  message_icon=Error  message=Power Supply Voltage Too Low
      settings: AttributesFormatString="\"%<message>\""  SourceProductName=QUARC Targets
  Show Message on Host1 : quarc_library/Sinks/Error Handling/Show Message on Host  message_type=Fixed error message  message_icon=Error  message=Power Supply Voltage Too High
      settings: AttributesFormatString="\"%<message>\""  SourceProductName=QUARC Targets
  Show Message on Host10 : quarc_library/Sinks/Error Handling/Show Message on Host  message_type=Fixed error message  message_icon=Error  message=Stepper Channel B Current Too High
      settings: AttributesFormatString="\"%<message>\""  SourceProductName=QUARC Targets
  Show Message on Host11 : quarc_library/Sinks/Error Handling/Show Message on Host  message_type=Fixed error message  message_icon=Error  message=Stepper Channel B Driver Over Current/Temperature
      settings: AttributesFormatString="\"%<message>\""  SourceProductName=QUARC Targets
  Show Message on Host12 : quarc_library/Sinks/Error Handling/Show Message on Host  message_type=Fixed error message  message_icon=Error  message=Stepper Channel A Driver Over Current/Temperature
      settings: AttributesFormatString="\"%<message>\""  SourceProductName=QUARC Targets
  Show Message on Host13 : quarc_library/Sinks/Error Handling/Show Message on Host  message_type=Fixed error message  message_icon=Error  message=Servo Motor Voltage Out of Range
      settings: AttributesFormatString="\"%<message>\""  SourceProductName=QUARC Targets
  Show Message on Host14 : quarc_library/Sinks/Error Handling/Show Message on Host  message_type=Fixed error message  message_icon=Error  message=Device Over-Temperature
      settings: AttributesFormatString="\"%<message>\""  SourceProductName=QUARC Targets
  Show Message on Host2 : quarc_library/Sinks/Error Handling/Show Message on Host  message_type=Fixed error message  message_icon=Error  message=Power Supply Current Too High
      settings: AttributesFormatString="\"%<message>\""  SourceProductName=QUARC Targets
  Show Message on Host3 : quarc_library/Sinks/Error Handling/Show Message on Host  message_type=Fixed error message  message_icon=Error  message=DC Motor Current Too High
      settings: AttributesFormatString="\"%<message>\""  SourceProductName=QUARC Targets
  Show Message on Host4 : quarc_library/Sinks/Error Handling/Show Message on Host  message_type=Fixed error message  message_icon=Error  message=DC Motor Driver Over Current/Temperature
      settings: AttributesFormatString="\"%<message>\""  SourceProductName=QUARC Targets
  Show Message on Host5 : quarc_library/Sinks/Error Handling/Show Message on Host  message_type=Fixed error message  message_icon=Error  message=Servo Motor Current Too High
      settings: AttributesFormatString="\"%<message>\""  SourceProductName=QUARC Targets
  Show Message on Host6 : quarc_library/Sinks/Error Handling/Show Message on Host  message_type=Fixed error message  message_icon=Error  message=BLDC Channel A Current Too High
      settings: AttributesFormatString="\"%<message>\""  SourceProductName=QUARC Targets
  Show Message on Host7 : quarc_library/Sinks/Error Handling/Show Message on Host  message_type=Fixed error message  message_icon=Error  message=BLDC Channel B Current Too High
      settings: AttributesFormatString="\"%<message>\""  SourceProductName=QUARC Targets
  Show Message on Host8 : quarc_library/Sinks/Error Handling/Show Message on Host  message_type=Fixed error message  message_icon=Error  message=BLDC Channel C Current Too High
      settings: AttributesFormatString="\"%<message>\""  SourceProductName=QUARC Targets
  Show Message on Host9 : quarc_library/Sinks/Error Handling/Show Message on Host  message_type=Fixed error message  message_icon=Error  message=Stepper Channel A Current Too High
      settings: AttributesFormatString="\"%<message>\""  SourceProductName=QUARC Targets
  wires:
  In1/1 -> Demux/1
  Demux/1 -> Show Message on Host/1
  Demux/2 -> Show Message on Host1/1
  Demux/3 -> Show Message on Host2/1
  Demux/4 -> Show Message on Host3/1
  Demux/5 -> Show Message on Host4/1
  Demux/6 -> Show Message on Host5/1
  Demux/8 -> Show Message on Host6/1
  Demux/9 -> Show Message on Host7/1
  Demux/10 -> Show Message on Host8/1
  Demux/11 -> Show Message on Host9/1
  Demux/12 -> Show Message on Host10/1
  Demux/13 -> Show Message on Host12/1
  Demux/14 -> Show Message on Host11/1
  Demux/15 -> Show Message on Host14/1
  Demux/7 -> Show Message on Host13/1

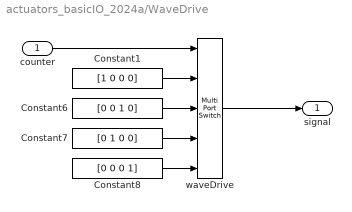
== system actuators_basicIO_2024a/WaveDrive ==
  counter : Inport
  Constant1 : Constant  Value=[1 0 0 0]
  Constant6 : Constant  Value=[0 0 1 0]
  Constant7 : Constant  Value=[0 1 0 0]
  Constant8 : Constant  Value=[0 0 0 1]
  waveDrive : MultiPortSwitch  Inputs=4  SaturateOnIntegerOverflow=off  InputSameDT=off
  signal : Outport
  wires:
  Constant6/1 -> waveDrive/3
  Constant7/1 -> waveDrive/4
  counter/1 -> waveDrive/1
  waveDrive/1 -> signal/1
  Constant8/1 -> waveDrive/5
  Constant1/1 -> waveDrive/2

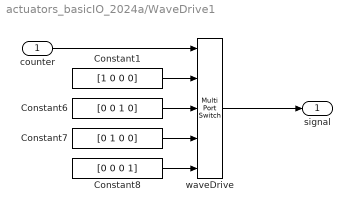
== system actuators_basicIO_2024a/WaveDrive1 ==
  counter : Inport
  Constant1 : Constant  Value=[1 0 0 0]
  Constant6 : Constant  Value=[0 0 1 0]
  Constant7 : Constant  Value=[0 1 0 0]
  Constant8 : Constant  Value=[0 0 0 1]
  waveDrive : MultiPortSwitch  Inputs=4  SaturateOnIntegerOverflow=off  InputSameDT=off
  signal : Outport
  wires:
  Constant6/1 -> waveDrive/3
  Constant7/1 -> waveDrive/4
  counter/1 -> waveDrive/1
  waveDrive/1 -> signal/1
  Constant8/1 -> waveDrive/5
  Constant1/1 -> waveDrive/2

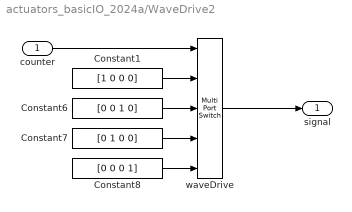
== system actuators_basicIO_2024a/WaveDrive2 ==
  counter : Inport
  Constant1 : Constant  Value=[1 0 0 0]
  Constant6 : Constant  Value=[0 0 1 0]
  Constant7 : Constant  Value=[0 1 0 0]
  Constant8 : Constant  Value=[0 0 0 1]
  waveDrive : MultiPortSwitch  Inputs=4  SaturateOnIntegerOverflow=off  InputSameDT=off
  signal : Outport
  wires:
  Constant6/1 -> waveDrive/3
  Constant7/1 -> waveDrive/4
  counter/1 -> waveDrive/1
  waveDrive/1 -> signal/1
  Constant8/1 -> waveDrive/5
  Constant1/1 -> waveDrive/2

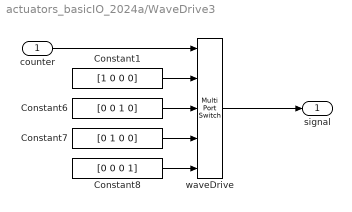
== system actuators_basicIO_2024a/WaveDrive3 ==
  counter : Inport
  Constant1 : Constant  Value=[1 0 0 0]
  Constant6 : Constant  Value=[0 0 1 0]
  Constant7 : Constant  Value=[0 1 0 0]
  Constant8 : Constant  Value=[0 0 0 1]
  waveDrive : MultiPortSwitch  Inputs=4  SaturateOnIntegerOverflow=off  InputSameDT=off
  signal : Outport
  wires:
  Constant6/1 -> waveDrive/3
  Constant7/1 -> waveDrive/4
  counter/1 -> waveDrive/1
  waveDrive/1 -> signal/1
  Constant8/1 -> waveDrive/5
  Constant1/1 -> waveDrive/2

== matlab function actuators_basicIO_2024a/MATLAB Function2 ==
  data: v input; pos output; neg output
function [pos, neg]= fcn(v)

if v >= 0
    pos = v;
    neg = 0;
else
    pos = 0;
    neg = abs(v);
end

== matlab function actuators_basicIO_2024a/MATLAB Function3 ==
  data: v input; pos output; neg output
function [pos, neg]= fcn(v)

if v >= 0
    pos = v;
    neg = 0;
else
    pos = 0;
    neg = abs(v);
end

== matlab function actuators_basicIO_2024a/MATLAB Function4 ==
  data: v input; pos output; neg output
function [pos, neg]= fcn(v)

if v >= 0
    pos = v;
    neg = 0;
else
    pos = 0;
    neg = abs(v);
end

== matlab function actuators_basicIO_2024a/MATLAB Function1 ==
  data: v input; pos output; neg output
function [pos, neg]= fcn(v)

if v >= 0
    pos = v;
    neg = 0;
else
    pos = 0;
    neg = abs(v);
end
